simulink model "ctrl_systems_2"  (Simulink 8.4)
settings: Solver=ode45  StartTime=0.0  StopTime=60  MaxStep=0.01  RelTol=1e-3
values from neighbouring files (symbols this model uses):
  A = XX    [codigo_Prac5.m]
  k = As*sqrt(2*g)    [codigo_Prac5.m]
  K = XX    [codigo_Prac5.m]
  T = tau    [codigo_Prac5.m]
  x0_ini = [2*XX  XX]    [codigo_Prac5.m]
settings Model: Creator=carles  LastModifiedBy=win04  CovHtmlReporting=off
settings DebuggingCC: FcnCallInpInsideContextMsg=EnableAllAsWarning  FrameProcessingCompatibilityMsg=error

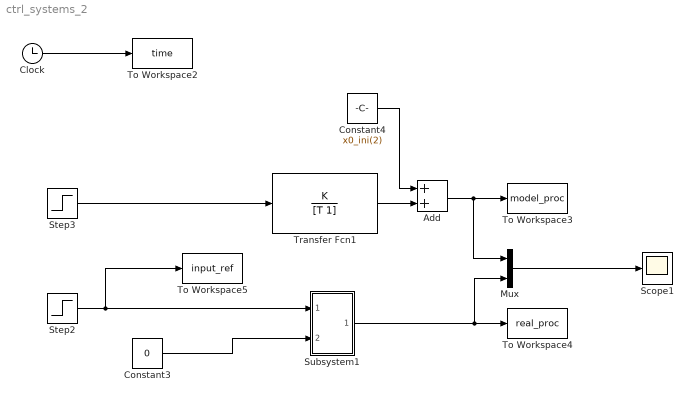
== system ctrl_systems_2 ==
  Add : Sum
  Clock : Clock
  Constant3 : Constant  Value=0
  Constant4 : Constant  Value=x0_ini(2)
  Mux : Mux  Inputs=2
  Scope1 : Scope
      settings: TimeRange=auto  LimitDataPoints=on  MaxDataPoints=5000  SaveToWorkspace=off  YMin=-0.00503  YMax=0.04586  SampleTime=-1
  Step2 : Step  Time=5  Before=2  After=2.5  SampleTime=0
  Step3 : Step  Time=5  After=0.5  SampleTime=0
  Subsystem1 : Subsystem
  To Workspace2 : ToWorkspace  VariableName=time  SampleTime=-1
  To Workspace3 : ToWorkspace  VariableName=model_proc  SampleTime=-1
  To Workspace4 : ToWorkspace  VariableName=real_proc  SampleTime=-1
  To Workspace5 : ToWorkspace  VariableName=input_ref  SaveFormat=Structure With Time  SampleTime=-1
  Transfer Fcn1 : TransferFcn  Numerator=K  Denominator=[T 1]
  wires:
  Step2/1 -> Subsystem1/1(In1), To Workspace5/1
  Constant3/1 -> Subsystem1/2(In2)
  Subsystem1/1(Out2) -> Mux/2, To Workspace4/1
  Mux/1 -> Scope1/1
  Step3/1 -> Transfer Fcn1/1
  Transfer Fcn1/1 -> Add/2
  Add/1 -> Mux/1, To Workspace3/1
  Constant4/1 -> Add/1
  Clock/1 -> To Workspace2/1

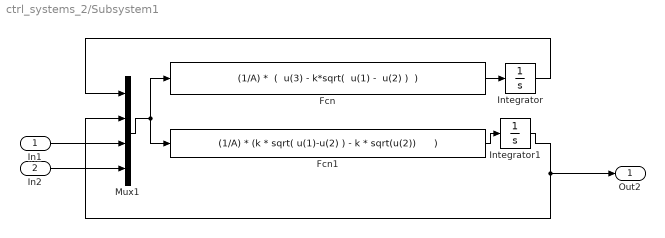
== system ctrl_systems_2/Subsystem1 ==
  In1 : Inport
  In2 : Inport  Port=2
  Fcn : Fcn  Expr="(1/A) *  (  u(3) - k*sqrt(  u(1) -  u(2) )  )"
  Fcn1 : Fcn  Expr="(1/A) * (k * sqrt( u(1)-u(2) ) - k * sqrt(u(2))      )"
  Integrator : Integrator  InitialCondition=x0_ini(1)
  Integrator1 : Integrator  InitialCondition=x0_ini(2)
  Mux1 : Mux
  Out2 : Outport
  wires:
  In1/1 -> Mux1/3
  In2/1 -> Mux1/4
  Integrator1/1 -> Out2/1, Mux1/2
  Integrator/1 -> Mux1/1
  Mux1/1 -> Fcn/1, Fcn1/1
  Fcn1/1 -> Integrator1/1
  Fcn/1 -> Integrator/1
